simulink model "demo_access_AP"  (R2015a)
settings: Solver=ode1  StartTime=0.0  StopTime=Inf  FixedStep=1/(62.5*4)  RelTol=1e-3
libraries: aerolibanimutils x2, instrumentlib x2
settings Model: Creator=Matt  LastModifiedBy=Matt
settings DataIOCC: SignalLoggingSaveFormat=ModelDataLogs
settings OptimizationCC: ExpressionDepthLimit=2147483647  OptimizeModelRefInitCode=on  LifeSpan=1
settings DebuggingCC: UnderspecifiedInitializationDetection=Classic  MergeDetectMultiDrivingBlocksExec=none  SolverPrmCheckMsg=warning  FcnCallInpInsideContextMsg=UseLocalSettings  StateNameClashWarn=warning
settings RTWCC: SystemTargetFile=ert.tlc  TemplateMakefile=ert_default_tmf  Description=Real-Time Workshop Embedded Coder
settings CodeAppCC: IgnoreCustomStorageClasses=off  CustomSymbolStrType=$N$R$M  InternalIdentifier=Classic
settings ERTTargetCC: ParMdlRefBuildCompliant=on  CompOptLevelCompliant=on  ConcurrentExecutionCompliant=on  ERTFirstTimeCompliant=on  SupportVariableSizeSignals=off  ModelStepFunctionPrototypeControlCompliant=on  CPPClassGenCompliant=on  InlinedParameterPlacement=Hierarchical  ERTCustomFileTemplate=example_file_process.tlc

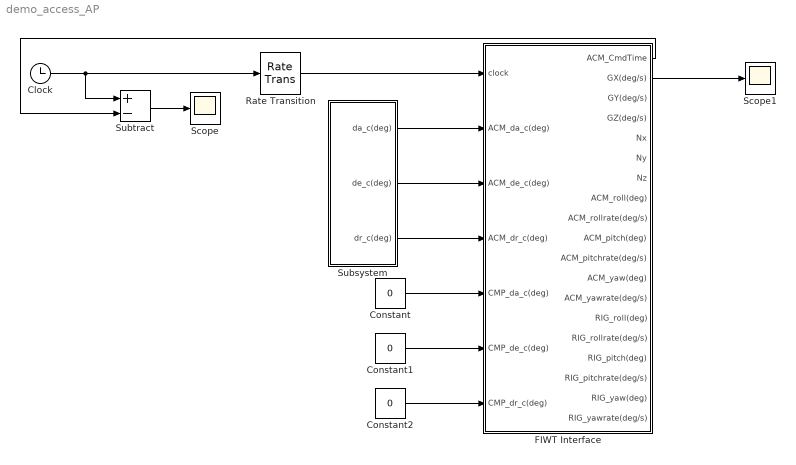
== system demo_access_AP ==
  Clock : Clock
      settings: Decimation=250
  Constant : Constant  Value=0
  Constant1 : Constant  Value=0
  Constant2 : Constant  Value=0
  FIWT Interface : Subsystem
  Rate Transition : RateTransition  OutPortSampleTime=1/62.5
  Scope : Scope
      settings: YMin=0.01  YMax=0.19
  Scope1 : Scope
      settings: YMin=-1  YMax=1
  Subsystem : Subsystem
  Subtract : Sum  Inputs=+-
  wires:
  Clock/1 -> Subtract/1, Rate Transition/1
  Subtract/1 -> Scope/1
  FIWT Interface/1(ACM_CmdTime) -> Subtract/2
  Constant/1 -> FIWT Interface/5(CMP_da_c(deg))
  Constant1/1 -> FIWT Interface/6(CMP_de_c(deg))
  Constant2/1 -> FIWT Interface/7(CMP_dr_c(deg))
  FIWT Interface/2(GX(deg/s)) -> Scope1/1
  Rate Transition/1 -> FIWT Interface/1(clock)
  Subsystem/1(da_c(deg)) -> FIWT Interface/2(ACM_da_c(deg))
  Subsystem/2(de_c(deg)) -> FIWT Interface/3(ACM_de_c(deg))
  Subsystem/3(dr_c(deg)) -> FIWT Interface/4(ACM_dr_c(deg))

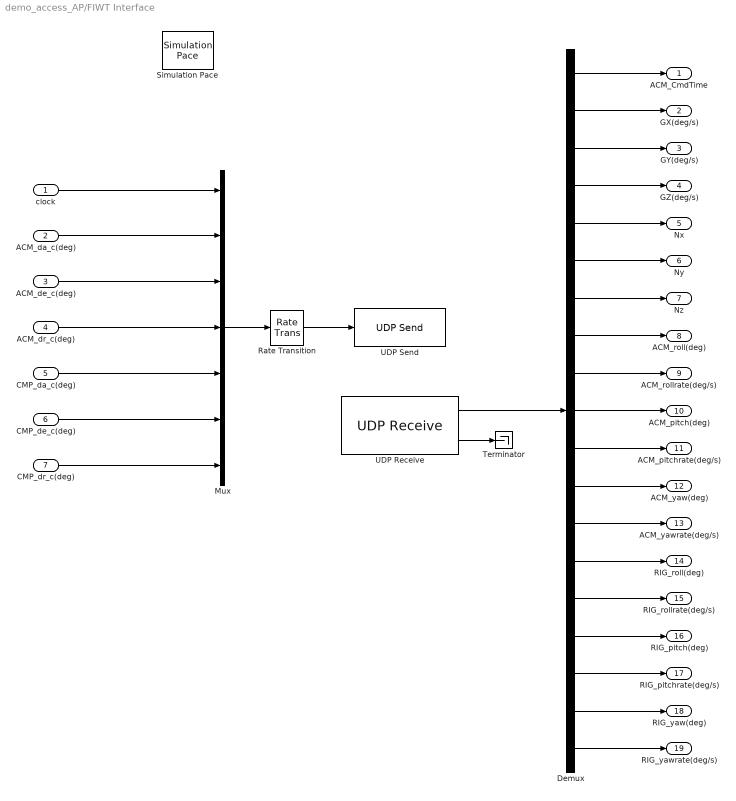
== system demo_access_AP/FIWT Interface ==
  clock : Inport
  ACM_da_c(deg) : Inport  Port=2
  ACM_de_c(deg) : Inport  Port=3
  ACM_dr_c(deg) : Inport  Port=4
  CMP_da_c(deg) : Inport  Port=5
  CMP_de_c(deg) : Inport  Port=6
  CMP_dr_c(deg) : Inport  Port=7
  Demux : Demux  Outputs=19
  Mux : Mux  Inputs=7
  Rate Transition : RateTransition  OutPortSampleTime=1/62.5
  Simulation Pace : aerolibanimutils/Simulation Pace  SimulationPace=1  SleepMode=MATLAB Thread  OutputPaceError=off  SampleTime=-1
      settings: AttributesFormatString=%<SimulationPace> sec/sec
  Terminator : Terminator
  UDP Receive : instrumentlib/UDP Receive  Priority=1  Host=127.0.0.1  Port=8080  LocalPort=8081  DataSize="[1  19]"  EnableBlockingMode=off  Timeout=1/250  SampleTime=-1  DataType=double  ByteOrder=BigEndian
  UDP Send : instrumentlib/UDP Send  Priority=3  Host=127.0.0.1  Port=9090  LocalPort=-1  EnableBlockingMode=on  ByteOrder=BigEndian
  ACM_CmdTime : Outport
  GX(deg/s) : Outport  Port=2
  GY(deg/s) : Outport  Port=3
  GZ(deg/s) : Outport  Port=4
  Nx : Outport  Port=5
  Ny : Outport  Port=6
  Nz : Outport  Port=7
  ACM_roll(deg) : Outport  Port=8
  ACM_rollrate(deg/s) : Outport  Port=9
  ACM_pitch(deg) : Outport  Port=10
  ACM_pitchrate(deg/s) : Outport  Port=11
  ACM_yaw(deg) : Outport  Port=12
  ACM_yawrate(deg/s) : Outport  Port=13
  RIG_roll(deg) : Outport  Port=14
  RIG_rollrate(deg/s) : Outport  Port=15
  RIG_pitch(deg) : Outport  Port=16
  RIG_pitchrate(deg/s) : Outport  Port=17
  RIG_yaw(deg) : Outport  Port=18
  RIG_yawrate(deg/s) : Outport  Port=19
  wires:
  Mux/1 -> Rate Transition/1
  Rate Transition/1 -> UDP Send/1
  UDP Receive/2 -> Terminator/1
  clock/1 -> Mux/1
  ACM_da_c(deg)/1 -> Mux/2
  UDP Receive/1 -> Demux/1
  Demux/1 -> ACM_CmdTime/1
  Demux/2 -> GX(deg/s)/1
  Demux/3 -> GY(deg/s)/1
  Demux/4 -> GZ(deg/s)/1
  Demux/5 -> Nx/1
  Demux/6 -> Ny/1
  Demux/7 -> Nz/1
  Demux/8 -> ACM_roll(deg)/1
  Demux/9 -> ACM_rollrate(deg/s)/1
  Demux/10 -> ACM_pitch(deg)/1
  Demux/11 -> ACM_pitchrate(deg/s)/1
  Demux/12 -> ACM_yaw(deg)/1
  Demux/13 -> ACM_yawrate(deg/s)/1
  Demux/14 -> RIG_roll(deg)/1
  Demux/15 -> RIG_rollrate(deg/s)/1
  Demux/16 -> RIG_pitch(deg)/1
  Demux/17 -> RIG_pitchrate(deg/s)/1
  Demux/18 -> RIG_yaw(deg)/1
  Demux/19 -> RIG_yawrate(deg/s)/1
  ACM_de_c(deg)/1 -> Mux/3
  ACM_dr_c(deg)/1 -> Mux/4
  CMP_da_c(deg)/1 -> Mux/5
  CMP_de_c(deg)/1 -> Mux/6
  CMP_dr_c(deg)/1 -> Mux/7

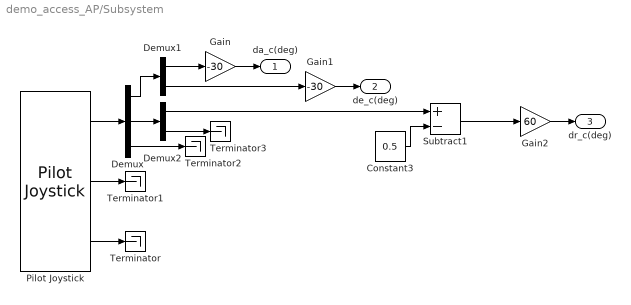
== system demo_access_AP/Subsystem ==
  Constant3 : Constant  Value=0.5
  Demux : Demux  Outputs=3
  Demux1 : Demux  Outputs=2
  Demux2 : Demux  Outputs=2
  Gain : Gain  Gain=-30
  Gain1 : Gain  Gain=-30
  Gain2 : Gain  Gain=60
  Pilot Joystick : aerolibanimutils/Pilot Joystick  JoystickID=Joystick1  OutputConfiguration=AllOutputs  SampleTime=1/62.5
  Subtract1 : Sum  Inputs=+-
  Terminator{,1..3} (4 alike) : Terminator
  da_c(deg) : Outport
  de_c(deg) : Outport  Port=2
  dr_c(deg) : Outport  Port=3
  wires:
  Pilot Joystick/1 -> Demux/1
  Demux/1 -> Demux1/1
  Demux1/1 -> Gain/1
  Demux1/2 -> Gain1/1
  Demux/2 -> Demux2/1
  Constant3/1 -> Subtract1/2
  Demux2/1 -> Subtract1/1
  Subtract1/1 -> Gain2/1
  Gain/1 -> da_c(deg)/1
  Gain1/1 -> de_c(deg)/1
  Gain2/1 -> dr_c(deg)/1
  Pilot Joystick/3 -> Terminator/1
  Pilot Joystick/2 -> Terminator1/1
  Demux/3 -> Terminator2/1
  Demux2/2 -> Terminator3/1
